simulink model "sim_HGO_test"  (R2017a)
settings: Solver=FixedStepAuto  StartTime=0.0  StopTime=10.0  FixedStep=simulation_step  RelTol=1e-3
values from neighbouring files (symbols this model uses):
  filter_pole = 30    [Init_HGO.m]
undefined symbols (not defined in the file or in its folder): control_step, Tb, TK, Tl1, Tl2, Tmu1, Tmu2
libraries: simulink x3
settings Model: Creator=ignacio  LastModifiedBy=ignacio

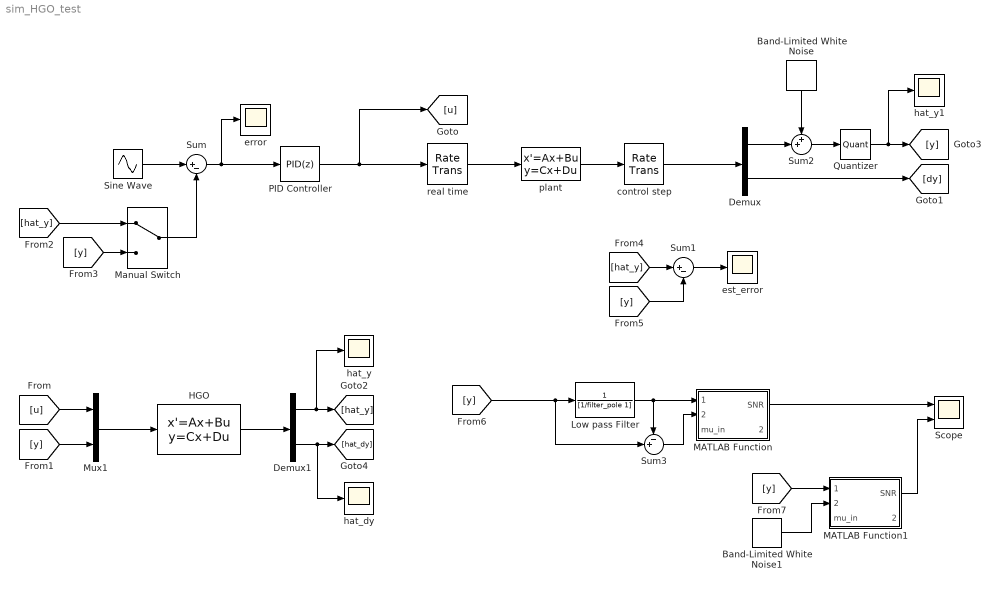
== system sim_HGO_test ==
  Band-Limited White Noise : simulink/Sources/Band-Limited White Noise  Cov=1e-8  Ts=control_step  seed=[23341]
  Band-Limited White Noise1 : simulink/Sources/Band-Limited White Noise  Cov=1e-8  Ts=control_step  seed=[23341]
  Demux : Demux  Outputs=2
  Demux1 : Demux  Outputs=2
  HGO : StateSpace  A=[0 1;0 0]-[1/Tmu1 0; 0 1/Tmu2^2]*[Tl1;Tl2]*[1 0]  B=[[0;1] [1/Tmu1 0; 0 1/Tmu2^2]*[Tl1;Tl2]]  C=eye(2)  D=zeros(2)  X0=[0 0]
  Low pass Filter : TransferFcn  Denominator=[1/filter_pole 1]
  MATLAB Function : MATLAB Function  TreatAsAtomicUnit=on
  MATLAB Function1 : MATLAB Function  TreatAsAtomicUnit=on
  Manual Switch : ManualSwitch
  Mux1 : Mux  Inputs=2
  PID Controller : simulink/Continuous/PID Controller  Controller=PID  TimeDomain=Discrete-time  SampleTime=control_step  IntegratorMethod=Forward Euler  FilterMethod=Forward Euler  Form=Parallel  UseFilter=on  ControllerParametersSource=internal  P=1092.89974140753  I=4384.73682138891  D=60.7835917377219  N=1569.69443157927  InitialConditionSource=internal  InitialConditionForIntegrator=0  InitialConditionForFilter=0  ExternalReset=none  LimitOutput=off  UpperSaturationLimit=inf  LowerSaturationLimit=-inf  LinearizeAsGain=on  AntiWindupMode=none  Kb=1  TrackingMode=off  Kt=1  PParamMin=[]  PParamMax=[]  IParamMin=[]  IParamMax=[]  DParamMin=[]  DParamMax=[]  NParamMin=[]  NParamMax=[]  KbParamMin=[]  KbParamMax=[]  KtParamMin=[]  KtParamMax=[]  POutMin=[]  POutMax=[]  IOutMin=[]  IOutMax=[]  DOutMin=[]  DOutMax=[]  NOutMin=[]  NOutMax=[]  KbOutMin=[]  KbOutMax=[]  KtOutMin=[]  KtOutMax=[]  IntegratorOutMin=[]  IntegratorOutMax=[]  FilterOutMin=[]  FilterOutMax=[]  SumOutMin=[]  SumOutMax=[]  SumI1OutMin=[]  SumI1OutMax=[]  SumI2OutMin=[]  SumI2OutMax=[]  SumI3OutMin=[]  SumI3OutMax=[]  SumDOutMin=[]  SumDOutMax=[]  SaturationOutMin=[]  SaturationOutMax=[]  IntegratorContinuousStateAttributes=''  IntegratorStateMustResolveToSignalObject=off  IntegratorRTWStateStorageClass=Auto  FilterContinuousStateAttributes=''  FilterStateMustResolveToSignalObject=off  FilterRTWStateStorageClass=Auto  DifferentiatorICPrevScaledInput=0  DifferentiatorOutMin=[]  DifferentiatorOutMax=[]  InitialConditionSetting=State (most efficient)
  Quantizer : Quantizer  QuantizationInterval=1e-3
  Scope : Scope  NumInputPorts=2
  Sine Wave : Sin  Frequency=2*pi*0.5  SampleTime=1e-3
  Sum : Sum  Inputs=|+-
  Sum1 : Sum  Inputs=|+-
  Sum2 : Sum  Inputs=++|
  Sum3 : Sum  Inputs=-+|
  control step : RateTransition  OutPortSampleTime=1e-3
  error : Scope
  est_error : Scope
  hat_dy : Scope
  hat_y : Scope
  hat_y1 : Scope
  plant : StateSpace  A=[0 1;-TK -Tb]  B=[0;1]  C=eye(2)  D=[0;0]  X0=[0 0]
  real time : RateTransition  OutPortSampleTime=simulation_step
  wires:
  Sine Wave/1 -> Sum/1
  Sum/1 -> error/1, PID Controller/1
  control step/1 -> Demux/1
  real time/1 -> plant/1
  PID Controller/1 -> [u], real time/1
  Sum2/1 -> Quantizer/1
  plant/1 -> control step/1
  Band-Limited White Noise/1 -> Sum2/1
  Demux/1 -> Sum2/2
  [u] -> Mux1/1
  Mux1/1 -> HGO/1
  HGO/1 -> Demux1/1
  Quantizer/1 -> hat_y1/1, [y]
  Demux/2 -> [dy]
  [y] -> Mux1/2
  Demux1/1 -> hat_y/1, [hat_y]
  Demux1/2 -> hat_dy/1, [hat_dy]
  [hat_y] -> Manual Switch/1
  [y] -> Manual Switch/2
  Manual Switch/1 -> Sum/2
  Sum1/1 -> est_error/1
  [hat_y] -> Sum1/1
  [y] -> Sum1/2
  [y] -> Sum3/2, Low pass Filter/1
  Low pass Filter/1 -> MATLAB Function/1(denoised_signal), Sum3/1
  Sum3/1 -> MATLAB Function/2(noise_signal)
  MATLAB Function/1(SNR) -> Scope/1
  [y] -> MATLAB Function1/1(denoised_signal)
  Band-Limited White Noise1/1 -> MATLAB Function1/2(noise_signal)
  MATLAB Function1/1(SNR) -> Scope/2

== matlab function sim_HGO_test/MATLAB Function1 ==
  data: denoised_signal input; noise_signal input; SNR output; mu_in input; mu_out output
function [SNR, mu_out] = fcn(denoised_signal,noise_signal, mu_in)
% Calculate signal Energy
% Obs.:Signal avg power would be Energy/Nsamples
    signalEn = rssq(denoised_signal).^2;
    noiseEn  = rssq(noise_signal).^2;
    
% Both energies have equal number of samples, therefore one doesn't need to
% calculate SNR as power
%--------------------------
% Calculate SNR
SNR = 10 * log10(signalEn ./ noiseEn);

%Condition for mu value update
if SNR > 20
    mu_out = mu_in;
else
    %mu_out = mu_in - 10^floor(log10(mu_in));
end

== matlab function sim_HGO_test/MATLAB Function ==
  data: denoised_signal input; noise_signal input; SNR output; mu_in input; mu_out output
function [SNR, mu_out] = fcn(denoised_signal,noise_signal, mu_in)
% Calculate signal Energy
% Obs.:Signal avg power would be Energy/Nsamples
    signalEn = rssq(denoised_signal).^2;
    noiseEn  = rssq(noise_signal).^2;
    
% Both energies have equal number of samples, therefore one doesn't need to
% calculate SNR as power
%--------------------------
% Calculate SNR
SNR = 10 * log10(signalEn ./ noiseEn);

%Condition for mu value update
if SNR > 20
    mu_out = mu_in;
else
    %mu_out = mu_in - 10^floor(log10(mu_in));
end
